simulink model "test"  (R2025b)
settings: Solver=VariableStepAuto  StartTime=0.0  StopTime=10.0  RelTol=1e-3
values from neighbouring files (symbols this model uses):
  amplituda = 2    [dane.m]
  b = 1    [dane.m]
  B = 2    [dane.m]
  Kp = 0.5    [dane.m]
  okres = 3    [dane.m]
  T = 0.3    [dane.m]
  Tp = 0.1    [dane.m]
libraries: simulink x1
settings Model: Creator=USER  LastModifiedBy=USER

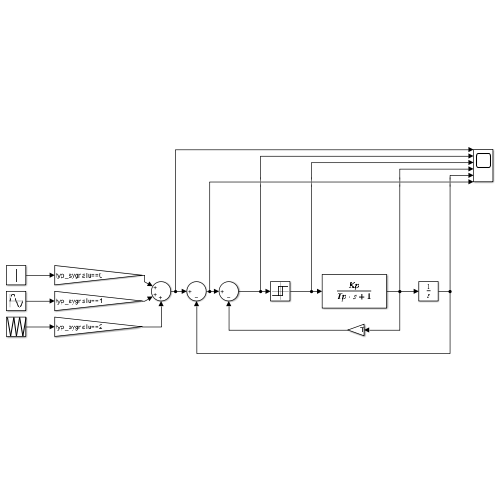
[thumbnail: Simulink's stored preview of the top-level diagram]
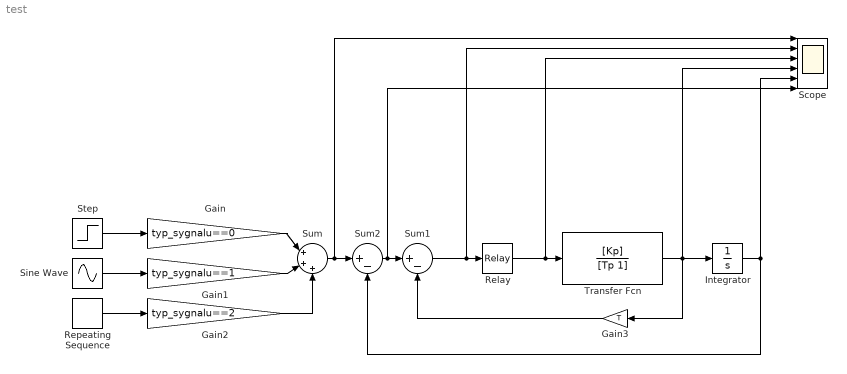
== system test ==
  Gain : Gain  Gain=typ_sygnalu==0
  Gain1 : Gain  Gain=typ_sygnalu==1
  Gain2 : Gain  Gain=typ_sygnalu==2
  Gain3 : Gain  Gain=T
  Integrator : Integrator
  Relay : Relay  OnSwitchValue=b  OffSwitchValue=-b  OnOutputValue=B  OffOutputValue=-B
  Repeating Sequence : simulink/Sources/Repeating Sequence  rep_seq_t=[0 okres/2 okres]  rep_seq_y=[amplituda -amplituda amplituda]
  Scope : Scope  NumInputPorts=6
      settings: ActiveDisplayYMinimum=-3.1057815348752458  ActiveDisplayYMaximum=4.9707783667898093
  Sine Wave : Sin  Amplitude=amplituda  Frequency=(1/okres)*(2*pi)  SampleTime=0
  Step : Step  Time=0  After=amplituda  SampleTime=0
  Sum : Sum  Inputs=|+++
  Sum1 : Sum  Inputs=|+-
  Sum2 : Sum  Inputs=|+-
  Transfer Fcn : TransferFcn  Numerator=[Kp]  Denominator=[Tp 1]
  wires:
  Repeating Sequence/1 -> Gain2/1
  Sine Wave/1 -> Gain1/1
  Step/1 -> Gain/1
  Gain/1 -> Sum/1
  Gain1/1 -> Sum/2
  Gain2/1 -> Sum/3
  Sum/1 -> Sum2/1, Scope/1
  Relay/1 -> Scope/3, Transfer Fcn/1
  Transfer Fcn/1 -> Gain3/1, Integrator/1, Scope/4
  Sum1/1 -> Scope/2, Relay/1
  Gain3/1 -> Sum1/2
  Sum2/1 -> Scope/6, Sum1/1
  Integrator/1 -> Sum2/2, Scope/5
